simulink model "dual_hall_discrete_eso"  (R2024b)
settings: Solver=FixedStepDiscrete  StartTime=0.0  StopTime=eso_t_stop_s  FixedStep=eso_Ts  RelTol=1e-3
model workspace (MAT data in the model file):
  eso_Ts = 0.0001
  eso_ab_alpha = 0.22
  eso_ab_beta = 0.018
  eso_angle_lpf_alpha = 0.975180456784
  eso_bandwidth_hz = 80
  eso_beta1 = 1507.96447372
  eso_beta2 = 757985.618004
  eso_beta3 = 127001709.283
  eso_initial_theta = -0.00107550784695
  eso_t_stop_s = 0.5
  eso_theta_meas_ts = timeseries
  eso_theta_meas_ts.Name = 'unnamed'
  eso_theta_meas_ts.DataInfo = tsdata.datametadata
  eso_theta_meas_ts.DataInfo.Interpolation = tsdata.interpolation
  eso_theta_meas_ts.DataInfo.Interpolation.Fhandle : function handle (value not decoded)
  eso_theta_meas_ts.DataInfo.Interpolation.Name = 'linear'
  eso_theta_meas_ts.TimeInfo = tsdata.timemetadata
  eso_theta_meas_ts.TimeInfo.Length = 5001
  eso_theta_meas_ts.TimeInfo.DuplicateTimes = 0
  eso_theta_meas_ts.TimeInfo.Time_ = [0 0.0001 0.0002 0.0003 0.0004 0.0005 0.0006 0.0007 0.0008 0.0009 0.001 0.0011 ... (5001 elements, 5001x1)]
  eso_theta_meas_ts.TimeInfo.Initialized = 1
  eso_theta_meas_ts.QualityInfo = tsdata.qualmetadata
  eso_theta_meas_ts.Data_ = [-0.00107550784695 0.00202512825295 0.00507032385874 0.00360222084162 0.0118127893328 0.00667152429571 0.0095162457883 0.00961245487541 0.00390759750929 0.00353130115901 0.00456286417416 0.0120582690606 ... (5001 elements, 5001x1)]
  eso_theta_true_ts = timeseries
  eso_theta_true_ts.Name = 'unnamed'
  eso_theta_true_ts.DataInfo = tsdata.datametadata
  eso_theta_true_ts.DataInfo.Interpolation = tsdata.interpolation
  eso_theta_true_ts.DataInfo.Interpolation.Fhandle : function handle (value not decoded)
  eso_theta_true_ts.DataInfo.Interpolation.Name = 'linear'
  eso_theta_true_ts.TimeInfo = tsdata.timemetadata
  eso_theta_true_ts.TimeInfo.Length = 5001
  eso_theta_true_ts.TimeInfo.DuplicateTimes = 0
  eso_theta_true_ts.TimeInfo.Time_ = [0 0.0001 0.0002 0.0003 0.0004 0.0005 0.0006 0.0007 0.0008 0.0009 0.001 0.0011 ... (5001 elements, 5001x1)]
  eso_theta_true_ts.TimeInfo.Initialized = 1
  eso_theta_true_ts.QualityInfo = tsdata.qualmetadata
  eso_theta_true_ts.Data_ = [0 0.0010471975512 0.00209439510239 0.00314159265359 0.00418879020479 0.00523598775598 0.00628318530718 0.00733038285838 0.00837758040957 0.00942477796077 0.010471975512 0.0115191730632 ... (5001 elements, 5001x1)]
settings Model: Creator=26683  LastModifiedBy=26683

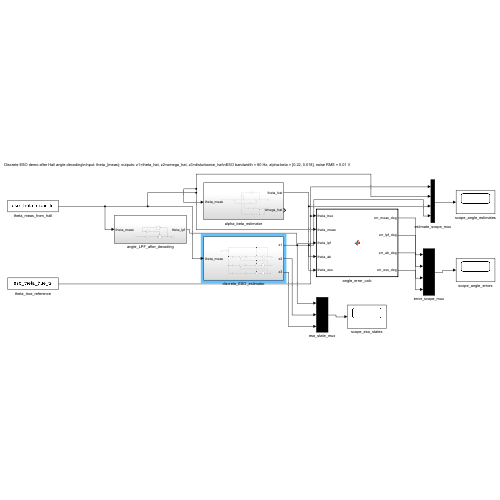
[thumbnail: Simulink's stored preview of the top-level diagram]
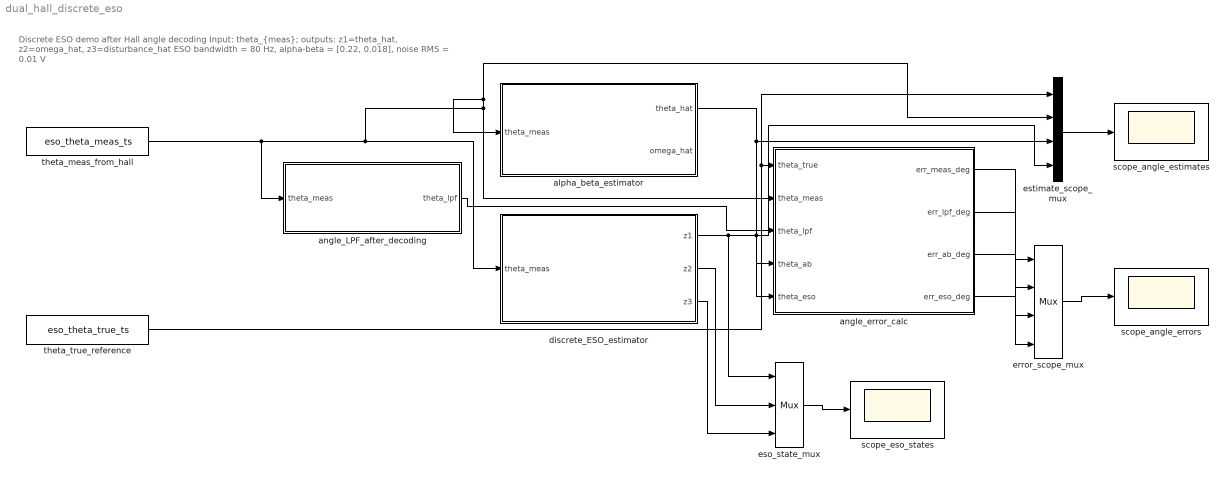
== system dual_hall_discrete_eso ==
  note: Discrete ESO demo after Hall angle decoding\nInput: theta_{meas}; outputs: z1=theta_hat, z2=omega_hat, z3=disturbance_hat\nESO bandwidth = 80 Hz, alpha-beta = [0.22, 0.018], noise RMS = 0.01 V
  alpha_beta_estimator : Subsystem
  angle_LPF_after_decoding : Subsystem
  angle_error_calc : MATLAB Function  TreatAsAtomicUnit=on
  discrete_ESO_estimator : Subsystem
  error_scope_mux : Mux
  eso_state_mux : Mux  Inputs=3
  estimate_scope_mux : Mux
  scope_angle_errors : Scope
  scope_angle_estimates : Scope
  scope_eso_states : Scope
  theta_meas_from_hall : FromWorkspace  VariableName=eso_theta_meas_ts
  theta_true_reference : FromWorkspace  VariableName=eso_theta_true_ts
  wires:
  theta_meas_from_hall/1 -> alpha_beta_estimator/1(theta_meas), estimate_scope_mux/2, angle_error_calc/2(theta_meas), discrete_ESO_estimator/1(theta_meas), angle_LPF_after_decoding/1(theta_meas)
  theta_true_reference/1 -> angle_error_calc/1(theta_true), estimate_scope_mux/1
  angle_LPF_after_decoding/1(theta_lpf) -> angle_error_calc/3(theta_lpf)
  alpha_beta_estimator/1(theta_hat) -> estimate_scope_mux/3, angle_error_calc/4(theta_ab)
  discrete_ESO_estimator/1(z1) -> angle_error_calc/5(theta_eso), estimate_scope_mux/4, eso_state_mux/1
  estimate_scope_mux/1 -> scope_angle_estimates/1
  angle_error_calc/1(err_meas_deg) -> error_scope_mux/1
  angle_error_calc/2(err_lpf_deg) -> error_scope_mux/2
  angle_error_calc/3(err_ab_deg) -> error_scope_mux/3
  angle_error_calc/4(err_eso_deg) -> error_scope_mux/4
  error_scope_mux/1 -> scope_angle_errors/1
  discrete_ESO_estimator/2(z2) -> eso_state_mux/2
  discrete_ESO_estimator/3(z3) -> eso_state_mux/3
  eso_state_mux/1 -> scope_eso_states/1

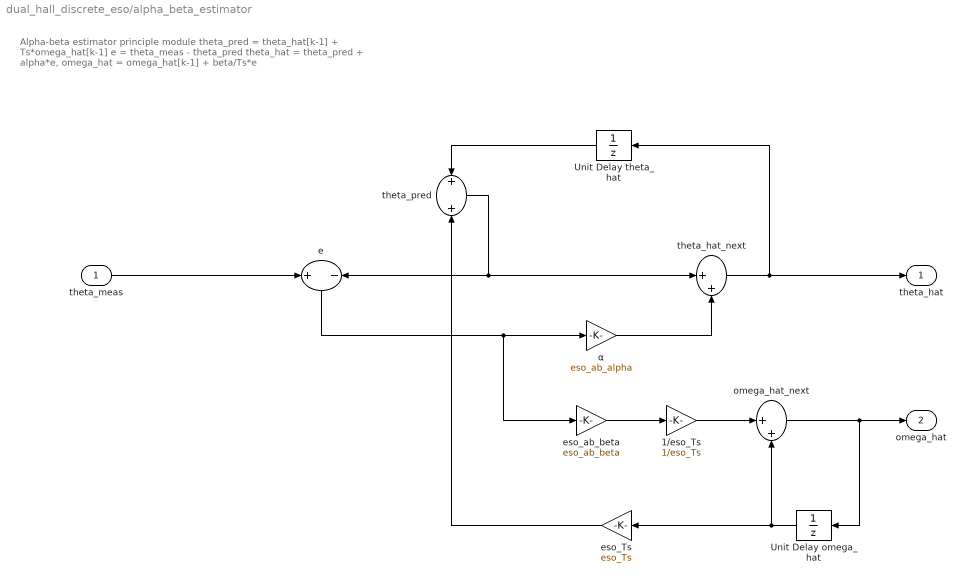
== system dual_hall_discrete_eso/alpha_beta_estimator ==
  note: Alpha-beta estimator principle module
      | theta_pred = theta_hat[k-1] + Ts*omega_hat[k-1]
      | e = theta_meas - theta_pred
      | theta_hat = theta_pred + alpha*e,  omega_hat = omega_hat[k-1] + beta/Ts*e
  theta_meas : Inport
  1/eso_Ts : Gain  Gain=1/eso_Ts
  Unit Delay omega_hat : UnitDelay  SampleTime=eso_Ts  HasFrameUpgradeWarning=on
  Unit Delay theta_hat : UnitDelay  InitialCondition=eso_initial_theta  SampleTime=eso_Ts  HasFrameUpgradeWarning=on
  "e " : Sum  Inputs=+|-
  eso_Ts : Gain  Gain=eso_Ts
  eso_ab_beta : Gain  Gain=eso_ab_beta
  omega_hat_next : Sum  Inputs=|++
  theta_hat_next : Sum  Inputs=|++
  theta_pred : Sum
  α : Gain  Gain=eso_ab_alpha
  theta_hat : Outport
  omega_hat : Outport  Port=2
  wires:
  Unit Delay omega_hat/1 -> eso_Ts/1, omega_hat_next/2
  theta_meas/1 -> "e "/1
  theta_pred/1 -> theta_hat_next/1, "e "/2
  "e "/1 -> eso_ab_beta/1, α/1
  theta_hat_next/1 -> Unit Delay theta_hat/1, theta_hat/1
  omega_hat_next/1 -> Unit Delay omega_hat/1, omega_hat/1
  Unit Delay theta_hat/1 -> theta_pred/1
  α/1 -> theta_hat_next/2
  eso_ab_beta/1 -> 1/eso_Ts/1
  eso_Ts/1 -> theta_pred/2
  1/eso_Ts/1 -> omega_hat_next/1

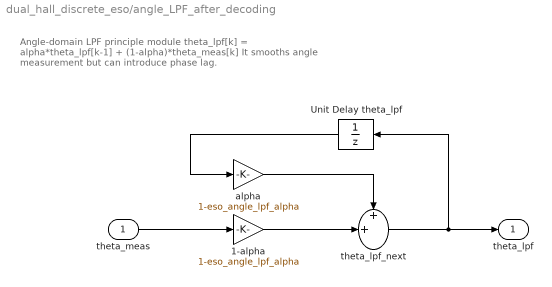
== system dual_hall_discrete_eso/angle_LPF_after_decoding ==
  note: Angle-domain LPF principle module
      | theta_lpf[k] = alpha*theta_lpf[k-1] + (1-alpha)*theta_meas[k]
      | It smooths angle measurement but can introduce phase lag.
  theta_meas : Inport
  1-alpha : Gain  Gain=1-eso_angle_lpf_alpha
  Unit Delay theta_lpf : UnitDelay  InitialCondition=eso_initial_theta  SampleTime=eso_Ts  HasFrameUpgradeWarning=on
  alpha : Gain  Gain=1-eso_angle_lpf_alpha
  theta_lpf_next : Sum  Inputs=++|
  theta_lpf : Outport
  wires:
  alpha/1 -> theta_lpf_next/1
  1-alpha/1 -> theta_lpf_next/2
  theta_lpf_next/1 -> theta_lpf/1, Unit Delay theta_lpf/1
  Unit Delay theta_lpf/1 -> alpha/1
  theta_meas/1 -> 1-alpha/1

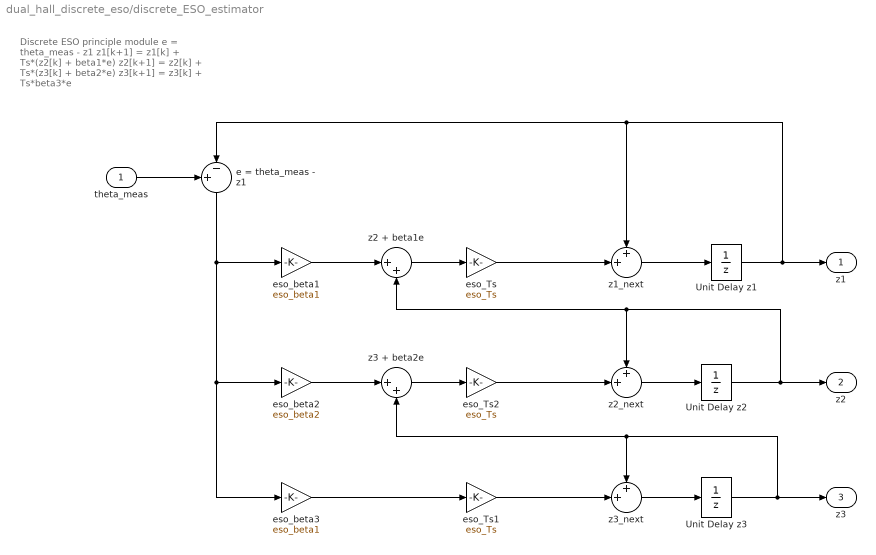
== system dual_hall_discrete_eso/discrete_ESO_estimator ==
  note: Discrete ESO principle module
      | e = theta_meas - z1
      | z1[k+1] = z1[k] + Ts*(z2[k] + beta1*e)
      | z2[k+1] = z2[k] + Ts*(z3[k] + beta2*e)
      | z3[k+1] = z3[k] + Ts*beta3*e
  theta_meas : Inport
  Unit Delay z1 : UnitDelay  InitialCondition=eso_initial_theta  SampleTime=eso_Ts  HasFrameUpgradeWarning=on
  Unit Delay z2 : UnitDelay  SampleTime=eso_Ts  HasFrameUpgradeWarning=on
  Unit Delay z3 : UnitDelay  SampleTime=eso_Ts  HasFrameUpgradeWarning=on
  e = theta_meas - z1 : Sum  Inputs=+-|
  eso_Ts : Gain  Gain=eso_Ts
  eso_Ts1 : Gain  Gain=eso_Ts
  eso_Ts2 : Gain  Gain=eso_Ts
  eso_beta1 : Gain  Gain=eso_beta1
  eso_beta2 : Gain  Gain=eso_beta2
  eso_beta3 : Gain  Gain=eso_beta1
  z1_next : Sum  Inputs=++|
  z2 + beta1e : Sum  Inputs=|++
  z2_next : Sum  Inputs=++|
  z3 + beta2e : Sum  Inputs=|++
  z3_next : Sum  Inputs=++|
  z1 : Outport
  z2 : Outport  Port=2
  z3 : Outport  Port=3
  wires:
  theta_meas/1 -> e = theta_meas - z1/1
  Unit Delay z1/1 -> e = theta_meas - z1/2, z1_next/1, z1/1
  e = theta_meas - z1/1 -> eso_beta3/1, eso_beta2/1, eso_beta1/1
  Unit Delay z2/1 -> z2 + beta1e/2, z2_next/1, z2/1
  Unit Delay z3/1 -> z3 + beta2e/2, z3_next/1, z3/1
  z2 + beta1e/1 -> eso_Ts/1
  z3 + beta2e/1 -> eso_Ts2/1
  eso_beta3/1 -> eso_Ts1/1
  eso_Ts/1 -> z1_next/2
  eso_Ts2/1 -> z2_next/2
  eso_Ts1/1 -> z3_next/2
  z1_next/1 -> Unit Delay z1/1
  z2_next/1 -> Unit Delay z2/1
  z3_next/1 -> Unit Delay z3/1
  eso_beta2/1 -> z3 + beta2e/1
  eso_beta1/1 -> z2 + beta1e/1

== matlab function dual_hall_discrete_eso/angle_error_calc ==
  data: theta_true input; err_meas_deg output; theta_meas input; theta_lpf input; theta_ab input; theta_eso input; err_lpf_deg output; err_ab_deg output; err_eso_deg output
function [err_meas_deg, err_lpf_deg, err_ab_deg, err_eso_deg] = f(theta_true, theta_meas, theta_lpf, theta_ab, theta_eso)
%#codegen
rad2deg_gain = 180/pi;
err_meas_deg = wrap_pi_local(theta_meas - theta_true)*rad2deg_gain;
err_lpf_deg = wrap_pi_local(theta_lpf - theta_true)*rad2deg_gain;
err_ab_deg = wrap_pi_local(theta_ab - theta_true)*rad2deg_gain;
err_eso_deg = wrap_pi_local(theta_eso - theta_true)*rad2deg_gain;
end

function y = wrap_pi_local(x)
y = mod(x + pi, 2*pi) - pi;
end
